simulink model "arvinpradipta_datadriver_modeling"  (R2023a)
settings: Solver=VariableStepAuto  StartTime=0.0  StopTime=10.0  RelTol=1e-3
values from neighbouring files (symbols this model uses):
  ts1 = 0.2    [mass_spring_damper_coding.slx.autosave.mat]
  ts2 = 0.5    [mass_spring_damper_coding.slx.autosave.mat]
settings Model: Creator=User  LastModifiedBy=User

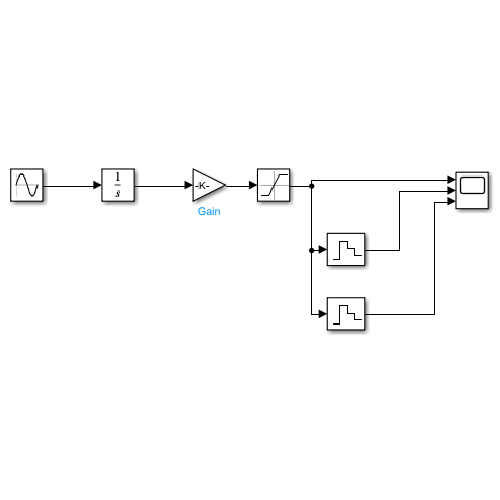
[thumbnail: Simulink's stored preview of the top-level diagram]
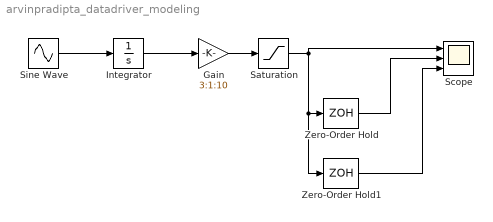
== system arvinpradipta_datadriver_modeling ==
  Gain : Gain  Gain=3:1:10
  Integrator : Integrator
  Saturation : Saturate  UpperLimit=rand(8,1)*10  LowerLimit=rand(8,1)*-10
  Scope : Scope  NumInputPorts=3
  Sine Wave : Sin  SampleTime=0
  Zero-Order Hold : ZeroOrderHold  SampleTime=ts1
  Zero-Order Hold1 : ZeroOrderHold  SampleTime=ts2
  wires:
  Zero-Order Hold/1 -> Scope/2
  Gain/1 -> Saturation/1
  Saturation/1 -> Zero-Order Hold1/1, Zero-Order Hold/1, Scope/1
  Sine Wave/1 -> Integrator/1
  Zero-Order Hold1/1 -> Scope/3
  Integrator/1 -> Gain/1
